simulink model "lateral1"  (Simulink 7.5)
settings: Solver=ode45  StartTime=0.0  StopTime=10.0  RelTol=1e-3
values from neighbouring files (symbols this model uses):
  ap = [Xu Xw 0 -g;Zu Zw Zq 0;Mu Mw Mq 0;0 0 1 0]    [gsnew2011.m]    (also in md11fla2011.m = [Xu Xw 0 -g 0;Zu Zw Zq 0 0;Mu Mw Mq 0 0;0 0 1 0 0;0 -1/U0  0)
  bp = [XL XT XR;ZL ZT ZR;ML MT MR;0 0 0]    [gsnew2011.m]    (also in md11fla2011.m = [XL XT XR;ZL ZT ZR;ML MT MR;0 0 0; 0 0 0])
  ncon = 3    [gsnew2011.m]    (also in md11fla2011.m)
  np = 4    [gsnew2011.m]    (also in md11fla2011.m = 5)
  pthrot = 0.6    [gsnew2011.m]    (also in md11fla2011.m = 1)
  Vc0 = 84.7    [gsnew2011.m]    (also in md11fla2011.m)
undefined symbols (not defined in the file or in its folder): alpha1L, K1l, K2l, R0
settings Model: Creator=knightofaccess  LastModifiedBy=knightofaccess

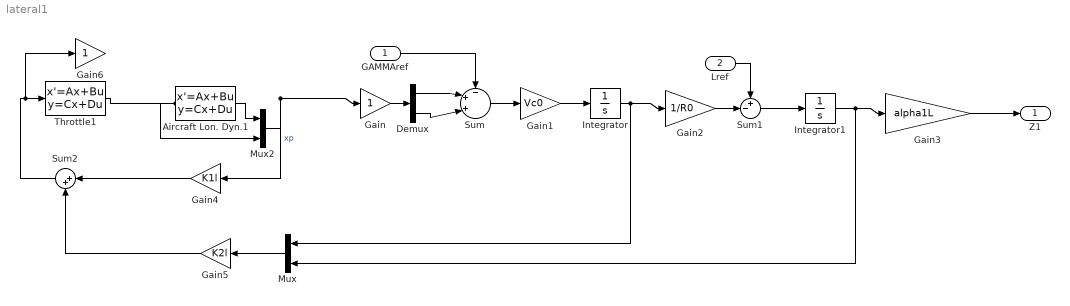
== system lateral1 ==
  GAMMAref : Inport  OutDataType=fixdt(1, 16)  OutScaling=2^0
  Lref : Inport  Port=2  OutDataType=fixdt(1, 16)  OutScaling=2^0
  Aircraft Lon. Dyn.1 : StateSpace  A=ap  B=bp  C=eye(np)  D=zeros(np,3)
  Demux : Demux  Outputs=2
  Gain : Gain  ParameterDataType=fixdt(1, 16)  ParameterScaling=2^0  OutDataType=fixdt(1, 16)  OutScaling=2^0
  Gain1 : Gain  Gain=Vc0  ParameterDataType=fixdt(1, 16)  ParameterScaling=2^0  OutDataType=fixdt(1, 16)  OutScaling=2^0
  Gain2 : Gain  Gain=1/R0  ParameterDataType=fixdt(1, 16)  ParameterScaling=2^0  OutDataType=fixdt(1, 16)  OutScaling=2^0
  Gain3 : Gain  Gain=alpha1L  ParameterDataType=fixdt(1, 16)  ParameterScaling=2^0  OutDataType=fixdt(1, 16)  OutScaling=2^0
  Gain4 : Gain  Gain=K1l  ParameterDataType=fixdt(1, 16)  ParameterScaling=2^0  OutDataType=fixdt(1, 16)  OutScaling=2^0
  Gain5 : Gain  Gain=K2l  ParameterDataType=fixdt(1, 16)  ParameterScaling=2^0  OutDataType=fixdt(1, 16)  OutScaling=2^0
  Gain6 : Gain  ParameterDataType=fixdt(1, 16)  ParameterScaling=2^0  OutDataType=fixdt(1, 16)  OutScaling=2^0
  Integrator : Integrator
  Integrator1 : Integrator
  Mux : Mux  Inputs=2
  Mux2 : Mux  Inputs=2
  Sum : Sum  Inputs=-++|  OutDataType=fixdt(1, 16)  OutScaling=2^0
  Sum1 : Sum  Inputs=+-|  OutDataType=fixdt(1, 16)  OutScaling=2^0
  Sum2 : Sum  Inputs=|++  OutDataType=fixdt(1, 16)  OutScaling=2^0
  Throttle1 : StateSpace  A=-pthrot*eye(ncon)  B=pthrot*eye(ncon)  C=eye(3)  D=zeros(3,3)
  Z1 : Outport  OutDataType=fixdt(1, 16)  OutScaling=2^0
  wires:
  Mux2/1 -> Gain/1, Gain4/1  "xp"
  Aircraft Lon. Dyn.1/1 -> Mux2/1
  Throttle1/1 -> Aircraft Lon. Dyn.1/1, Mux2/2
  Gain/1 -> Demux/1
  Demux/2 -> Sum/3
  Demux/1 -> Sum/2
  GAMMAref/1 -> Sum/1
  Sum/1 -> Gain1/1
  Gain1/1 -> Integrator/1
  Integrator/1 -> Gain2/1, Mux/1
  Gain2/1 -> Sum1/2
  Lref/1 -> Sum1/1
  Sum1/1 -> Integrator1/1
  Integrator1/1 -> Gain3/1, Mux/2
  Gain3/1 -> Z1/1
  Mux/1 -> Gain5/1
  Gain4/1 -> Sum2/1
  Gain5/1 -> Sum2/2
  Sum2/1 -> Throttle1/1, Gain6/1
